simulink library "outp"  (R2021b)
(part 11 of 11)

  VTPM_WriteChkLFID_raw/1 -> VTPM_WriteChkLFID_raw_Inproc/1  "VTPM_WriteChkLFID_raw"
  VTPM_WriteChkLFID_raw_Inproc/1 -> UnitConverter899/1
  UnitConverter899/1 -> VOUTP_WriteChkLFID_raw/1  "VOUTP_WriteChkLFID_raw"
  VTPM_WriteChkRFID_raw/1 -> VTPM_WriteChkRFID_raw_Inproc/1  "VTPM_WriteChkRFID_raw"
  VTPM_WriteChkRFID_raw_Inproc/1 -> UnitConverter900/1
  UnitConverter900/1 -> VOUTP_WriteChkRFID_raw/1  "VOUTP_WriteChkRFID_raw"
  VTPM_WriteChkLRID_raw/1 -> VTPM_WriteChkLRID_raw_Inproc/1  "VTPM_WriteChkLRID_raw"
  VTPM_WriteChkLRID_raw_Inproc/1 -> UnitConverter901/1
  UnitConverter901/1 -> VOUTP_WriteChkLRID_raw/1  "VOUTP_WriteChkLRID_raw"
  VTPM_WriteChkRRID_raw/1 -> VTPM_WriteChkRRID_raw_Inproc/1  "VTPM_WriteChkRRID_raw"
  VTPM_WriteChkRRID_raw_Inproc/1 -> UnitConverter902/1
  UnitConverter902/1 -> VOUTP_WriteChkRRID_raw/1  "VOUTP_WriteChkRRID_raw"
  VTPM_WriteChkfinLFID_raw/1 -> VTPM_WriteChkfinLFID_raw_Inproc/1  "VTPM_WriteChkfinLFID_raw"
  VTPM_WriteChkfinLFID_raw_Inproc/1 -> UnitConverter903/1
  UnitConverter903/1 -> VOUTP_WriteChkfinLFID_raw/1  "VOUTP_WriteChkfinLFID_raw"
  VTPM_WriteChkfinRFID_raw/1 -> VTPM_WriteChkfinRFID_raw_Inproc/1  "VTPM_WriteChkfinRFID_raw"
  VTPM_WriteChkfinRFID_raw_Inproc/1 -> UnitConverter904/1
  UnitConverter904/1 -> VOUTP_WriteChkfinRFID_raw/1  "VOUTP_WriteChkfinRFID_raw"
  VTPM_WriteChkfinLRID_raw/1 -> VTPM_WriteChkfinLRID_raw_Inproc/1  "VTPM_WriteChkfinLRID_raw"
  VTPM_WriteChkfinLRID_raw_Inproc/1 -> UnitConverter905/1
  UnitConverter905/1 -> VOUTP_WriteChkfinLRID_raw/1  "VOUTP_WriteChkfinLRID_raw"
  VTPM_WriteChkfinRRID_raw/1 -> VTPM_WriteChkfinRRID_raw_Inproc/1  "VTPM_WriteChkfinRRID_raw"
  VTPM_WriteChkfinRRID_raw_Inproc/1 -> UnitConverter906/1
  UnitConverter906/1 -> VOUTP_WriteChkfinRRID_raw/1  "VOUTP_WriteChkfinRRID_raw"
  VTPM_Flashchkdatavalid_enum/1 -> VTPM_Flashchkdatavalid_enum_Inproc/1  "VTPM_Flashchkdatavalid_enum"
  VTPM_Flashchkdatavalid_enum_Inproc/1 -> UnitConverter907/1
  UnitConverter907/1 -> VOUTP_Flashchkdatavalid_enum/1  "VOUTP_Flashchkdatavalid_enum"
  VTPM_Flashdatavalid_enum/1 -> VTPM_Flashdatavalid_enum_Inproc/1  "VTPM_Flashdatavalid_enum"
  VTPM_Flashdatavalid_enum_Inproc/1 -> UnitConverter908/1
  UnitConverter908/1 -> VOUTP_Flashdatavalid_enum/1  "VOUTP_Flashdatavalid_enum"
  VTPM_unlearnSfali_flg/1 -> VTPM_unlearnSfali_flg_Inproc/1  "VTPM_unlearnSfali_flg"
  VTPM_unlearnSfali_flg_Inproc/1 -> UnitConverter909/1
  UnitConverter909/1 -> VOUTP_unlearnSfali_flg/1  "VOUTP_unlearnSfali_flg"
  VTPM_unlearnSfailvalid_enum/1 -> VTPM_unlearnSfailvalid_enum_Inproc/1  "VTPM_unlearnSfailvalid_enum"
  VTPM_unlearnSfailvalid_enum_Inproc/1 -> UnitConverter910/1
  UnitConverter910/1 -> VOUTP_unlearnSfailvalid_enum/1  "VOUTP_unlearnSfailvalid_enum"
  VTPM_Prepresstempvalid_enum/1 -> VTPM_Prepresstempvalid_enum_Inproc/1  "VTPM_Prepresstempvalid_enum"
  VTPM_Prepresstempvalid_enum_Inproc/1 -> UnitConverter911/1
  UnitConverter911/1 -> VOUTP_Prepresstempvalid_enum/1  "VOUTP_Prepresstempvalid_enum"
  VTPM_FlashS1ID_raw/1 -> VTPM_FlashS1ID_raw_Inproc/1  "VTPM_FlashS1ID_raw"
  VTPM_FlashS1ID_raw_Inproc/1 -> UnitConverter912/1
  UnitConverter912/1 -> VOUTP_FlashS1ID_raw/1  "VOUTP_FlashS1ID_raw"
  VTPM_FlashS2ID_raw/1 -> VTPM_FlashS2ID_raw_Inproc/1  "VTPM_FlashS2ID_raw"
  VTPM_FlashS2ID_raw_Inproc/1 -> UnitConverter913/1
  UnitConverter913/1 -> VOUTP_FlashS2ID_raw/1  "VOUTP_FlashS2ID_raw"
  VTPM_FlashS3ID_raw/1 -> VTPM_FlashS3ID_raw_Inproc/1  "VTPM_FlashS3ID_raw"
  VTPM_FlashS3ID_raw_Inproc/1 -> UnitConverter914/1
  UnitConverter914/1 -> VOUTP_FlashS3ID_raw/1  "VOUTP_FlashS3ID_raw"
  VTPM_FlashS4ID_raw/1 -> VTPM_FlashS4ID_raw_Inproc/1  "VTPM_FlashS4ID_raw"
  VTPM_FlashS4ID_raw_Inproc/1 -> UnitConverter915/1
  UnitConverter915/1 -> VOUTP_FlashS4ID_raw/1  "VOUTP_FlashS4ID_raw"
  VTPM_FlashIDvalid_enum/1 -> VTPM_FlashIDvalid_enum_Inproc/1  "VTPM_FlashIDvalid_enum"
  VTPM_FlashIDvalid_enum_Inproc/1 -> UnitConverter916/1
  UnitConverter916/1 -> VOUTP_FlashIDvalid_enum/1  "VOUTP_FlashIDvalid_enum"
  VTPM_WritingCnt_enum/1 -> VTPM_WritingCnt_enum_Inproc/1  "VTPM_WritingCnt_enum"
  VTPM_WritingCnt_enum_Inproc/1 -> UnitConverter917/1
  UnitConverter917/1 -> VOUTP_WritingCnt_enum/1  "VOUTP_WritingCnt_enum"
  VTPM_TPMSTLCmd_flg/1 -> VTPM_TPMSTLCmd_flg_Inproc/1  "VTPM_TPMSTLCmd_flg"
  VTPM_TPMSTLCmd_flg_Inproc/1 -> UnitConverter918/1
  UnitConverter918/1 -> VOUTP_TPMSTLCmd_flg/1  "VOUTP_TPMSTLCmd_flg"
  VTPM_LProgress_enum/1 -> VTPM_LProgress_enum_Inproc/1  "VTPM_LProgress_enum"
  VTPM_LProgress_enum_Inproc/1 -> UnitConverter919/1
  UnitConverter919/1 -> VOUTP_LProgress_enum/1  "VOUTP_LProgress_enum"
  VTPM_TPMSSensorIDRegStart_flg/1 -> VTPM_TPMSSensorIDRegStart_flg_Inproc/1  "VTPM_TPMSSensorIDRegStart_flg"
  VTPM_TPMSSensorIDRegStart_flg_Inproc/1 -> UnitConverter920/1
  UnitConverter920/1 -> VOUTP_TPMSSensorIDRegStart_flg/1  "VOUTP_TPMSSensorIDRegStart_flg"
  VTPM_ModelVersion_raw/1 -> VTPM_ModelVersion_raw_Inproc/1  "VTPM_ModelVersion_raw"
  VTPM_ModelVersion_raw_Inproc/1 -> UnitConverter921/1
  UnitConverter921/1 -> VOUTP_ModelVersion_raw/1  "VOUTP_ModelVersion_raw"
  VTPM_ModelVersionChksum_raw/1 -> VTPM_ModelVersionChksum_raw_Inproc/1  "VTPM_ModelVersionChksum_raw"
  VTPM_ModelVersionChksum_raw_Inproc/1 -> UnitConverter922/1
  UnitConverter922/1 -> VOUTP_ModelVersionChksum_raw/1  "VOUTP_ModelVersionChksum_raw"
  VTQD_ParkRequest_flg/1 -> VTQD_ParkRequest_flg_Inproc/1  "VTQD_ParkRequest_flg"
  VTQD_ParkRequest_flg_Inproc/1 -> UnitConverter923/1
  UnitConverter923/1 -> VOUTP_ParkRequest_flg/1  "VOUTP_ParkRequest_flg"
  VTQD_TqSourceFr_enum/1 -> VTQD_TqSourceFr_enum_Inproc/1  "VTQD_TqSourceFr_enum"
  VTQD_TqSourceFr_enum_Inproc/1 -> UnitConverter924/1
  UnitConverter924/1 -> VOUTP_TqSourceFr_enum/1  "VOUTP_TqSourceFr_enum"
  VTQD_TqSourceRr_enum/1 -> VTQD_TqSourceRr_enum_Inproc/1  "VTQD_TqSourceRr_enum"
  VTQD_TqSourceRr_enum_Inproc/1 -> UnitConverter925/1
  UnitConverter925/1 -> VOUTP_TqSourceRr_enum/1  "VOUTP_TqSourceRr_enum"
  VTQD_FrEDUAvailBrkRgnTq_Nm/1 -> VTQD_FrEDUAvailBrkRgnTq_Nm_Inproc/1  "VTQD_FrEDUAvailBrkRgnTq_Nm"
  VTQD_FrEDUAvailBrkRgnTq_Nm_Inproc/1 -> UnitConverter926/1
  UnitConverter926/1 -> VOUTP_FrEDUAvailBrkRgnTq_Nm/1  "VOUTP_FrEDUAvailBrkRgnTq_Nm"
  VTQD_RrEDUAvailBrkRgnTq_Nm/1 -> VTQD_RrEDUAvailBrkRgnTq_Nm_Inproc/1  "VTQD_RrEDUAvailBrkRgnTq_Nm"
  VTQD_RrEDUAvailBrkRgnTq_Nm_Inproc/1 -> UnitConverter927/1
  UnitConverter927/1 -> VOUTP_RrEDUAvailBrkRgnTq_Nm/1  "VOUTP_RrEDUAvailBrkRgnTq_Nm"
  VTQD_EVDriveMode_enum/1 -> VTQD_EVDriveMode_enum_Inproc/1  "VTQD_EVDriveMode_enum"
  VTQD_EVDriveMode_enum_Inproc/1 -> UnitConverter928/1
  UnitConverter928/1 -> VOUTP_EVDriveMode_enum/1  "VOUTP_EVDriveMode_enum"
  VTQD_ShiftGearPosn_enum/1 -> VTQD_ShiftGearPosn_enum_Inproc/1  "VTQD_ShiftGearPosn_enum"
  VTQD_ShiftGearPosn_enum_Inproc/1 -> UnitConverter929/1
  UnitConverter929/1 -> VOUTP_ShiftGearPosn_enum/1  "VOUTP_ShiftGearPosn_enum"
  VTQD_PButtonSta_enum/1 -> VTQD_PButtonSta_enum_Inproc/1  "VTQD_PButtonSta_enum"
  VTQD_PButtonSta_enum_Inproc/1 -> UnitConverter930/1
  UnitConverter930/1 -> VOUTP_PButtonSta_enum/1  "VOUTP_PButtonSta_enum"
  VTQD_FrActvDmpDisabReq_flg/1 -> VTQD_FrActvDmpDisabReq_flg_Inproc/1  "VTQD_FrActvDmpDisabReq_flg"
  VTQD_FrActvDmpDisabReq_flg_Inproc/1 -> UnitConverter931/1
  UnitConverter931/1 -> VOUTP_FrActvDmpDisabReq_flg/1  "VOUTP_FrActvDmpDisabReq_flg"
  VTQD_RrActvDmpDisabReq_flg/1 -> VTQD_RrActvDmpDisabReq_flg_Inproc/1  "VTQD_RrActvDmpDisabReq_flg"
  VTQD_RrActvDmpDisabReq_flg_Inproc/1 -> UnitConverter932/1
  UnitConverter932/1 -> VOUTP_RrActvDmpDisabReq_flg/1  "VOUTP_RrActvDmpDisabReq_flg"
  VTQD_FrRgnDecrSta_flg/1 -> VTQD_FrRgnDecrSta_flg_Inproc/1  "VTQD_FrRgnDecrSta_flg"
  VTQD_FrRgnDecrSta_flg_Inproc/1 -> UnitConverter933/1
  UnitConverter933/1 -> VOUTP_FrRgnDecrSta_flg/1  "VOUTP_FrRgnDecrSta_flg"
  VTQD_RrRgnDecrSta_flg/1 -> VTQD_RrRgnDecrSta_flg_Inproc/1  "VTQD_RrRgnDecrSta_flg"
  VTQD_RrRgnDecrSta_flg_Inproc/1 -> UnitConverter934/1
  UnitConverter934/1 -> VOUTP_RrRgnDecrSta_flg/1  "VOUTP_RrRgnDecrSta_flg"
  VTQD_DriverWhlTqDemFr_Nm/1 -> VTQD_DriverWhlTqDemFr_Nm_Inproc/1  "VTQD_DriverWhlTqDemFr_Nm"
  VTQD_DriverWhlTqDemFr_Nm_Inproc/1 -> UnitConverter935/1
  UnitConverter935/1 -> VOUTP_DriverWhlTqDemFr_Nm/1  "VOUTP_DriverWhlTqDemFr_Nm"
  VTQD_DriverWhlTqDemRr_Nm/1 -> VTQD_DriverWhlTqDemRr_Nm_Inproc/1  "VTQD_DriverWhlTqDemRr_Nm"
  VTQD_DriverWhlTqDemRr_Nm_Inproc/1 -> UnitConverter936/1
  UnitConverter936/1 -> VOUTP_DriverWhlTqDemRr_Nm/1  "VOUTP_DriverWhlTqDemRr_Nm"
  VTQD_FrEDUActTq_Nm/1 -> VTQD_FrEDUActTq_Nm_Inproc/1  "VTQD_FrEDUActTq_Nm"
  VTQD_FrEDUActTq_Nm_Inproc/1 -> UnitConverter937/1
  UnitConverter937/1 -> VOUTP_FrEDUActTq_Nm/1  "VOUTP_FrEDUActTq_Nm"
  VTQD_RrEDUActTq_Nm/1 -> VTQD_RrEDUActTq_Nm_Inproc/1  "VTQD_RrEDUActTq_Nm"
  VTQD_RrEDUActTq_Nm_Inproc/1 -> UnitConverter938/1
  UnitConverter938/1 -> VOUTP_RrEDUActTq_Nm/1  "VOUTP_RrEDUActTq_Nm"
  VTQD_FrEDURolRgnTq_Nm/1 -> VTQD_FrEDURolRgnTq_Nm_Inproc/1  "VTQD_FrEDURolRgnTq_Nm"
  VTQD_FrEDURolRgnTq_Nm_Inproc/1 -> UnitConverter939/1
  UnitConverter939/1 -> VOUTP_FrEDURolRgnTq_Nm/1  "VOUTP_FrEDURolRgnTq_Nm"
  VTQD_RrEDURolRgnTq_Nm/1 -> VTQD_RrEDURolRgnTq_Nm_Inproc/1  "VTQD_RrEDURolRgnTq_Nm"
  VTQD_RrEDURolRgnTq_Nm_Inproc/1 -> UnitConverter940/1
  UnitConverter940/1 -> VOUTP_RrEDURolRgnTq_Nm/1  "VOUTP_RrEDURolRgnTq_Nm"
  VTQD_FrEDUSpd_rpm/1 -> VTQD_FrEDUSpd_rpm_Inproc/1  "VTQD_FrEDUSpd_rpm"
  VTQD_FrEDUSpd_rpm_Inproc/1 -> UnitConverter941/1
  UnitConverter941/1 -> VOUTP_FrEDUSpd_rpm/1  "VOUTP_FrEDUSpd_rpm"
  VTQD_RrEDUSpd_rpm/1 -> VTQD_RrEDUSpd_rpm_Inproc/1  "VTQD_RrEDUSpd_rpm"
  VTQD_RrEDUSpd_rpm_Inproc/1 -> UnitConverter942/1
  UnitConverter942/1 -> VOUTP_RrEDUSpd_rpm/1  "VOUTP_RrEDUSpd_rpm"
  VTQD_FrEDUSpdValid_flg/1 -> VTQD_FrEDUSpdValid_flg_Inproc/1  "VTQD_FrEDUSpdValid_flg"
  VTQD_FrEDUSpdValid_flg_Inproc/1 -> UnitConverter943/1
  UnitConverter943/1 -> VOUTP_FrEDUSpdValid_flg/1  "VOUTP_FrEDUSpdValid_flg"
  VTQD_FrEDUAvailBrkRgnTqV_flg/1 -> VTQD_FrEDUAvailBrkRgnTqV_flg_Inproc/1  "VTQD_FrEDUAvailBrkRgnTqV_flg"
  VTQD_FrEDUAvailBrkRgnTqV_flg_Inproc/1 -> UnitConverter944/1
  UnitConverter944/1 -> VOUTP_FrEDUAvailBrkRgnTqV_flg/1  "VOUTP_FrEDUAvailBrkRgnTqV_flg"
  VTQD_RrEDUSpdValid_flg/1 -> VTQD_RrEDUSpdValid_flg_Inproc/1  "VTQD_RrEDUSpdValid_flg"
  VTQD_RrEDUSpdValid_flg_Inproc/1 -> UnitConverter945/1
  UnitConverter945/1 -> VOUTP_RrEDUSpdValid_flg/1  "VOUTP_RrEDUSpdValid_flg"
  VTQD_RrEDUAvailBrkRgnTqV_flg/1 -> VTQD_RrEDUAvailBrkRgnTqV_flg_Inproc/1  "VTQD_RrEDUAvailBrkRgnTqV_flg"
  VTQD_RrEDUAvailBrkRgnTqV_flg_Inproc/1 -> UnitConverter946/1
  UnitConverter946/1 -> VOUTP_RrEDUAvailBrkRgnTqV_flg/1  "VOUTP_RrEDUAvailBrkRgnTqV_flg"
  VTQD_RgnAbnorSta_flg/1 -> VTQD_RgnAbnorSta_flg_Inproc/1  "VTQD_RgnAbnorSta_flg"
  VTQD_RgnAbnorSta_flg_Inproc/1 -> UnitConverter947/1
  UnitConverter947/1 -> VOUTP_RgnAbnorSta_flg/1  "VOUTP_RgnAbnorSta_flg"
  VTQD_PTCSPermSta_flg/1 -> VTQD_PTCSPermSta_flg_Inproc/1  "VTQD_PTCSPermSta_flg"
  VTQD_PTCSPermSta_flg_Inproc/1 -> UnitConverter948/1
  UnitConverter948/1 -> VOUTP_PTCSPermSta_flg/1  "VOUTP_PTCSPermSta_flg"
  VTQD_FrRgnPermSta_flg/1 -> VTQD_FrRgnPermSta_flg_Inproc/1  "VTQD_FrRgnPermSta_flg"
  VTQD_FrRgnPermSta_flg_Inproc/1 -> UnitConverter949/1
  UnitConverter949/1 -> VOUTP_FrRgnPermSta_flg/1  "VOUTP_FrRgnPermSta_flg"
  VTQD_RrRgnPermSta_flg/1 -> VTQD_RrRgnPermSta_flg_Inproc/1  "VTQD_RrRgnPermSta_flg"
  VTQD_RrRgnPermSta_flg_Inproc/1 -> UnitConverter950/1
  UnitConverter950/1 -> VOUTP_RrRgnPermSta_flg/1  "VOUTP_RrRgnPermSta_flg"
  VTQD_FrIdcMin_A/1 -> VTQD_FrIdcMin_A_Inproc/1  "VTQD_FrIdcMin_A"
  VTQD_FrIdcMin_A_Inproc/1 -> UnitConverter951/1
  UnitConverter951/1 -> VOUTP_FrIdcMin_A/1  "VOUTP_FrIdcMin_A"
  VTQD_FrIdcMax_A/1 -> VTQD_FrIdcMax_A_Inproc/1  "VTQD_FrIdcMax_A"
  VTQD_FrIdcMax_A_Inproc/1 -> UnitConverter952/1
  UnitConverter952/1 -> VOUTP_FrIdcMax_A/1  "VOUTP_FrIdcMax_A"
  VTQD_FrUdcMin_V/1 -> VTQD_FrUdcMin_V_Inproc/1  "VTQD_FrUdcMin_V"
  VTQD_FrUdcMin_V_Inproc/1 -> UnitConverter953/1
  UnitConverter953/1 -> VOUTP_FrUdcMin_V/1  "VOUTP_FrUdcMin_V"
  VTQD_FrUdcMax_V/1 -> VTQD_FrUdcMax_V_Inproc/1  "VTQD_FrUdcMax_V"
  VTQD_FrUdcMax_V_Inproc/1 -> UnitConverter954/1
  UnitConverter954/1 -> VOUTP_FrUdcMax_V/1  "VOUTP_FrUdcMax_V"
  VTQD_RrIdcMin_A/1 -> VTQD_RrIdcMin_A_Inproc/1  "VTQD_RrIdcMin_A"
  VTQD_RrIdcMin_A_Inproc/1 -> UnitConverter955/1
  UnitConverter955/1 -> VOUTP_RrIdcMin_A/1  "VOUTP_RrIdcMin_A"
  VTQD_RrIdcMax_A/1 -> VTQD_RrIdcMax_A_Inproc/1  "VTQD_RrIdcMax_A"
  VTQD_RrIdcMax_A_Inproc/1 -> UnitConverter956/1
  UnitConverter956/1 -> VOUTP_RrIdcMax_A/1  "VOUTP_RrIdcMax_A"
  VTQD_RrUdcMin_V/1 -> VTQD_RrUdcMin_V_Inproc/1  "VTQD_RrUdcMin_V"
  VTQD_RrUdcMin_V_Inproc/1 -> UnitConverter957/1
  UnitConverter957/1 -> VOUTP_RrUdcMin_V/1  "VOUTP_RrUdcMin_V"
  VTQD_RrUdcMax_V/1 -> VTQD_RrUdcMax_V_Inproc/1  "VTQD_RrUdcMax_V"
  VTQD_RrUdcMax_V_Inproc/1 -> UnitConverter958/1
  UnitConverter958/1 -> VOUTP_RrUdcMax_V/1  "VOUTP_RrUdcMax_V"
  VTQD_ReBrakeLPReq_flg/1 -> VTQD_ReBrakeLPReq_flg_Inproc/1  "VTQD_ReBrakeLPReq_flg"
  VTQD_ReBrakeLPReq_flg_Inproc/1 -> UnitConverter959/1
  UnitConverter959/1 -> VOUTP_ReBrakeLPReq_flg/1  "VOUTP_ReBrakeLPReq_flg"
  VTQD_CreepON_flg/1 -> VTQD_CreepON_flg_Inproc/1  "VTQD_CreepON_flg"
  VTQD_CreepON_flg_Inproc/1 -> UnitConverter960/1
  UnitConverter960/1 -> VOUTP_CreepON_flg/1  "VOUTP_CreepON_flg"
  VTQD_EquivAccPedalSWSta_flg/1 -> VTQD_EquivAccPedalSWSta_flg_Inproc/1  "VTQD_EquivAccPedalSWSta_flg"
  VTQD_EquivAccPedalSWSta_flg_Inproc/1 -> UnitConverter961/1
  UnitConverter961/1 -> VOUTP_EquivAccPedalSWSta_flg/1  "VOUTP_EquivAccPedalSWSta_flg"
  VTQD_DriveProtEn_flg/1 -> VTQD_DriveProtEn_flg_Inproc/1  "VTQD_DriveProtEn_flg"
  VTQD_DriveProtEn_flg_Inproc/1 -> UnitConverter962/1
  UnitConverter962/1 -> VOUTP_DriveProtEn_flg/1  "VOUTP_DriveProtEn_flg"
  VTQD_ActParkRequest_flg/1 -> VTQD_ActParkRequest_flg_Inproc/1  "VTQD_ActParkRequest_flg"
  VTQD_ActParkRequest_flg_Inproc/1 -> UnitConverter963/1
  UnitConverter963/1 -> VOUTP_ActParkRequest_flg/1  "VOUTP_ActParkRequest_flg"
  VTQD_IVIPwrLockSta_enum/1 -> VTQD_IVIPwrLockSta_enum_Inproc/1  "VTQD_IVIPwrLockSta_enum"
  VTQD_IVIPwrLockSta_enum_Inproc/1 -> UnitConverter964/1
  UnitConverter964/1 -> VOUTP_IVIPwrLockSta_enum/1  "VOUTP_IVIPwrLockSta_enum"
  VTQD_OPDHoldLamp_flg/1 -> VTQD_OPDHoldLamp_flg_Inproc/1  "VTQD_OPDHoldLamp_flg"
  VTQD_OPDHoldLamp_flg_Inproc/1 -> UnitConverter965/1
  UnitConverter965/1 -> VOUTP_OPDHoldLamp_flg/1  "VOUTP_OPDHoldLamp_flg"
  VTQD_SaveRegenMode_enum/1 -> VTQD_SaveRegenMode_enum_Inproc/1  "VTQD_SaveRegenMode_enum"
  VTQD_SaveRegenMode_enum_Inproc/1 -> UnitConverter966/1
  UnitConverter966/1 -> VOUTP_SaveRegenMode_enum/1  "VOUTP_SaveRegenMode_enum"
  VTQD_FDCVCURegenMode_enum/1 -> VTQD_FDCVCURegenMode_enum_Inproc/1  "VTQD_FDCVCURegenMode_enum"
  VTQD_FDCVCURegenMode_enum_Inproc/1 -> UnitConverter967/1
  UnitConverter967/1 -> VOUTP_FDCVCURegenMode_enum/1  "VOUTP_FDCVCURegenMode_enum"
  VTQD_SpdCtrlMode_enum/1 -> VTQD_SpdCtrlMode_enum_Inproc/1  "VTQD_SpdCtrlMode_enum"
  VTQD_SpdCtrlMode_enum_Inproc/1 -> UnitConverter968/1
  UnitConverter968/1 -> VOUTP_SpdCtrlMode_enum/1  "VOUTP_SpdCtrlMode_enum"
  VTQD_SpdCtrlSta_flg/1 -> VTQD_SpdCtrlSta_flg_Inproc/1  "VTQD_SpdCtrlSta_flg"
  VTQD_SpdCtrlSta_flg_Inproc/1 -> UnitConverter969/1
  UnitConverter969/1 -> VOUTP_SpdCtrlSta_flg/1  "VOUTP_SpdCtrlSta_flg"
  VTQD_SetSpd_kph/1 -> VTQD_SetSpd_kph_Inproc/1  "VTQD_SetSpd_kph"
  VTQD_SetSpd_kph_Inproc/1 -> UnitConverter970/1
  UnitConverter970/1 -> VOUTP_SetSpd_kph/1  "VOUTP_SetSpd_kph"
  VTQD_VehActSpd_kph/1 -> VTQD_VehActSpd_kph_Inproc/1  "VTQD_VehActSpd_kph"
  VTQD_VehActSpd_kph_Inproc/1 -> UnitConverter971/1
  UnitConverter971/1 -> VOUTP_VehActSpd_kph/1  "VOUTP_VehActSpd_kph"
  VTQD_RegenLimIndSta_flg/1 -> VTQD_RegenLimIndSta_flg_Inproc/1  "VTQD_RegenLimIndSta_flg"
  VTQD_RegenLimIndSta_flg_Inproc/1 -> UnitConverter972/1
  UnitConverter972/1 -> VOUTP_RegenLimIndSta_flg/1  "VOUTP_RegenLimIndSta_flg"
  VTQD_SetSpdLimWarn_flg/1 -> VTQD_SetSpdLimWarn_flg_Inproc/1  "VTQD_SetSpdLimWarn_flg"
  VTQD_SetSpdLimWarn_flg_Inproc/1 -> UnitConverter973/1
  UnitConverter973/1 -> VOUTP_SetSpdLimWarn_flg/1  "VOUTP_SetSpdLimWarn_flg"
  VTQR_FrTMTqReq_Nm/1 -> VTQR_FrTMTqReq_Nm_Inproc/1  "VTQR_FrTMTqReq_Nm"
  VTQR_FrTMTqReq_Nm_Inproc/1 -> UnitConverter974/1
  UnitConverter974/1 -> VOUTP_FrTMTqReq_Nm/1  "VOUTP_FrTMTqReq_Nm"
  VTQR_RrTMTqReq_Nm/1 -> VTQR_RrTMTqReq_Nm_Inproc/1  "VTQR_RrTMTqReq_Nm"
  VTQR_RrTMTqReq_Nm_Inproc/1 -> UnitConverter975/1
  UnitConverter975/1 -> VOUTP_RrTMTqReq_Nm/1  "VOUTP_RrTMTqReq_Nm"
  VV2L_ReqOBCV2LEna_enum/1 -> VV2L_ReqOBCV2LEna_enum_Inproc/1  "VV2L_ReqOBCV2LEna_enum"
  VV2L_ReqOBCV2LEna_enum_Inproc/1 -> UnitConverter976/1
  UnitConverter976/1 -> VOUTP_ReqOBCV2LEna_enum/1  "VOUTP_ReqOBCV2LEna_enum"
  VV2L_ReqV2LIVIPopup_enum/1 -> VV2L_ReqV2LIVIPopup_enum_Inproc/1  "VV2L_ReqV2LIVIPopup_enum"
  VV2L_ReqV2LIVIPopup_enum_Inproc/1 -> UnitConverter977/1
  UnitConverter977/1 -> VOUTP_ReqV2LIVIPopup_enum/1  "VOUTP_ReqV2LIVIPopup_enum"
  VV2L_ReqV2LIVIDisChrg_enum/1 -> VV2L_ReqV2LIVIDisChrg_enum_Inproc/1  "VV2L_ReqV2LIVIDisChrg_enum"
  VV2L_ReqV2LIVIDisChrg_enum_Inproc/1 -> UnitConverter978/1
  UnitConverter978/1 -> VOUTP_ReqV2LIVIDisChrg_enum/1  "VOUTP_ReqV2LIVIDisChrg_enum"
  VV2L_ReqOBCExtrV2LEna_enum/1 -> VV2L_ReqOBCExtrV2LEna_enum_Inproc/1  "VV2L_ReqOBCExtrV2LEna_enum"
  VV2L_ReqOBCExtrV2LEna_enum_Inproc/1 -> UnitConverter979/1
  UnitConverter979/1 -> VOUTP_ReqOBCExtrV2LEna_enum/1  "VOUTP_ReqOBCExtrV2LEna_enum"
  VV2L_ReqOBCIntrV2LEna_enum/1 -> VV2L_ReqOBCIntrV2LEna_enum_Inproc/1  "VV2L_ReqOBCIntrV2LEna_enum"
  VV2L_ReqOBCIntrV2LEna_enum_Inproc/1 -> UnitConverter980/1
  UnitConverter980/1 -> VOUTP_ReqOBCIntrV2LEna_enum/1  "VOUTP_ReqOBCIntrV2LEna_enum"
  VV2L_HVPO120VGrpALDSt_enum/1 -> VV2L_HVPO120VGrpALDSt_enum_Inproc/1  "VV2L_HVPO120VGrpALDSt_enum"
  VV2L_HVPO120VGrpALDSt_enum_Inproc/1 -> UnitConverter981/1
  UnitConverter981/1 -> VOUTP_HVPO120VGrpALDSt_enum/1  "VOUTP_HVPO120VGrpALDSt_enum"
  VV2L_HVPO120VGrpBLDSt_enum/1 -> VV2L_HVPO120VGrpBLDSt_enum_Inproc/1  "VV2L_HVPO120VGrpBLDSt_enum"
  VV2L_HVPO120VGrpBLDSt_enum_Inproc/1 -> UnitConverter982/1
  UnitConverter982/1 -> VOUTP_HVPO120VGrpBLDSt_enum/1  "VOUTP_HVPO120VGrpBLDSt_enum"
  VVMC_FeatSetSpdFinal_raw32/1 -> VVMC_FeatSetSpdFinal_raw32_Inproc/1  "VVMC_FeatSetSpdFinal_raw32"
  VVMC_FeatSetSpdFinal_raw32_Inproc/1 -> UnitConverter983/1
  UnitConverter983/1 -> VOUTP_FeatSetSpdFinal_raw32/1  "VOUTP_FeatSetSpdFinal_raw32"
  VVMC_VehicleSpeed_mph/1 -> VVMC_VehicleSpeed_mph_Inproc/1  "VVMC_VehicleSpeed_mph"
  VVMC_VehicleSpeed_mph_Inproc/1 -> UnitConverter984/1
  UnitConverter984/1 -> VOUTP_VehicleSpeed_mph/1  "VOUTP_VehicleSpeed_mph"
  VVMC_VehicleSpeed_kph/1 -> VVMC_VehicleSpeed_kph_Inproc/1  "VVMC_VehicleSpeed_kph"
  VVMC_VehicleSpeed_kph_Inproc/1 -> UnitConverter985/1
  UnitConverter985/1 -> VOUTP_VehicleSpeed_kph/1  "VOUTP_VehicleSpeed_kph"
  VVMC_MeterIndSpeed_raw32/1 -> VVMC_MeterIndSpeed_raw32_Inproc/1  "VVMC_MeterIndSpeed_raw32"
  VVMC_MeterIndSpeed_raw32_Inproc/1 -> UnitConverter986/1
  UnitConverter986/1 -> VOUTP_MeterIndSpeed_raw32/1  "VOUTP_MeterIndSpeed_raw32"
  VVMC_VMCAEBCtrlAvail_flg/1 -> VVMC_VMCAEBCtrlAvail_flg_Inproc/1  "VVMC_VMCAEBCtrlAvail_flg"
  VVMC_VMCAEBCtrlAvail_flg_Inproc/1 -> UnitConverter987/1
  UnitConverter987/1 -> VOUTP_VMCAEBCtrlAvail_flg/1  "VOUTP_VMCAEBCtrlAvail_flg"
  VVMC_VMCACCCtrlAvail_flg/1 -> VVMC_VMCACCCtrlAvail_flg_Inproc/1  "VVMC_VMCACCCtrlAvail_flg"
  VVMC_VMCACCCtrlAvail_flg_Inproc/1 -> UnitConverter988/1
  UnitConverter988/1 -> VOUTP_VMCACCCtrlAvail_flg/1  "VOUTP_VMCACCCtrlAvail_flg"
  VVMC_VMCCCCtrlAvail_flg/1 -> VVMC_VMCCCCtrlAvail_flg_Inproc/1  "VVMC_VMCCCCtrlAvail_flg"
  VVMC_VMCCCCtrlAvail_flg_Inproc/1 -> UnitConverter989/1
  UnitConverter989/1 -> VOUTP_VMCCCCtrlAvail_flg/1  "VOUTP_VMCCCCtrlAvail_flg"
  VVMC_VMCMSACtrlAvail_flg/1 -> VVMC_VMCMSACtrlAvail_flg_Inproc/1  "VVMC_VMCMSACtrlAvail_flg"
  VVMC_VMCMSACtrlAvail_flg_Inproc/1 -> UnitConverter990/1
  UnitConverter990/1 -> VOUTP_VMCMSACtrlAvail_flg/1  "VOUTP_VMCMSACtrlAvail_flg"
  VVMC_FeatArbitrSta_enum/1 -> VVMC_FeatArbitrSta_enum_Inproc/1  "VVMC_FeatArbitrSta_enum"
  VVMC_FeatArbitrSta_enum_Inproc/1 -> UnitConverter991/1
  UnitConverter991/1 -> VOUTP_FeatArbitrSta_enum/1  "VOUTP_FeatArbitrSta_enum"
  VVMC_FeatReqSpd_kph/1 -> VVMC_FeatReqSpd_kph_Inproc/1  "VVMC_FeatReqSpd_kph"
  VVMC_FeatReqSpd_kph_Inproc/1 -> UnitConverter992/1
  UnitConverter992/1 -> VOUTP_FeatReqSpd_kph/1  "VOUTP_FeatReqSpd_kph"
  VVMC_JerkPCT_pct/1 -> VVMC_JerkPCT_pct_Inproc/1  "VVMC_JerkPCT_pct"
  VVMC_JerkPCT_pct_Inproc/1 -> UnitConverter993/1
  UnitConverter993/1 -> VOUTP_JerkPCT_pct/1  "VOUTP_JerkPCT_pct"
  VVMC_LimitPCT_pct/1 -> VVMC_LimitPCT_pct_Inproc/1  "VVMC_LimitPCT_pct"
  VVMC_LimitPCT_pct_Inproc/1 -> UnitConverter994/1
  UnitConverter994/1 -> VOUTP_LimitPCT_pct/1  "VOUTP_LimitPCT_pct"
  VVMC_FrontRearSlipRatioCtrl_flg/1 -> VVMC_FrontRearSlipRatioCtrl_flg_Inproc/1  "VVMC_FrontRearSlipRatioCtrl_flg"
  VVMC_FrontRearSlipRatioCtrl_flg_Inproc/1 -> UnitConverter995/1
  UnitConverter995/1 -> VOUTP_FrontRearSlipRatioCtrl_flg/1  "VOUTP_FrontRearSlipRatioCtrl_flg"
  VVMC_RearWhlSlipRatioCtrl_flg/1 -> VVMC_RearWhlSlipRatioCtrl_flg_Inproc/1  "VVMC_RearWhlSlipRatioCtrl_flg"
  VVMC_RearWhlSlipRatioCtrl_flg_Inproc/1 -> UnitConverter996/1
  UnitConverter996/1 -> VOUTP_RearWhlSlipRatioCtrl_flg/1  "VOUTP_RearWhlSlipRatioCtrl_flg"
  VVMC_SingleWhlSlipRatioCtrl_flg/1 -> VVMC_SingleWhlSlipRatioCtrl_flg_Inproc/1  "VVMC_SingleWhlSlipRatioCtrl_flg"
  VVMC_SingleWhlSlipRatioCtrl_flg_Inproc/1 -> UnitConverter997/1
  UnitConverter997/1 -> VOUTP_SingleWhlSlipRatioCtrl_flg/1  "VOUTP_SingleWhlSlipRatioCtrl_flg"
  VVMC_LatAccCtrl_flg/1 -> VVMC_LatAccCtrl_flg_Inproc/1  "VVMC_LatAccCtrl_flg"
  VVMC_LatAccCtrl_flg_Inproc/1 -> UnitConverter998/1
  UnitConverter998/1 -> VOUTP_LatAccCtrl_flg/1  "VOUTP_LatAccCtrl_flg"
  VVMC_SafetyCtrl_flg/1 -> VVMC_SafetyCtrl_flg_Inproc/1  "VVMC_SafetyCtrl_flg"
  VVMC_SafetyCtrl_flg_Inproc/1 -> UnitConverter999/1
  UnitConverter999/1 -> VOUTP_SafetyCtrl_flg/1  "VOUTP_SafetyCtrl_flg"
  VVMC_SPD2ACCAct_flg/1 -> VVMC_SPD2ACCAct_flg_Inproc/1  "VVMC_SPD2ACCAct_flg"
  VVMC_SPD2ACCAct_flg_Inproc/1 -> UnitConverter1000/1
  UnitConverter1000/1 -> VOUTP_SPD2ACCAct_flg/1  "VOUTP_SPD2ACCAct_flg"
  VVMC_AccCalcuPID_mps2/1 -> VVMC_AccCalcuPID_mps2_Inproc/1  "VVMC_AccCalcuPID_mps2"
  VVMC_AccCalcuPID_mps2_Inproc/1 -> UnitConverter1001/1
  UnitConverter1001/1 -> VOUTP_AccCalcuPID_mps2/1  "VOUTP_AccCalcuPID_mps2"
  VVMC_ISOAccLimit_mps2/1 -> VVMC_ISOAccLimit_mps2_Inproc/1  "VVMC_ISOAccLimit_mps2"
  VVMC_ISOAccLimit_mps2_Inproc/1 -> UnitConverter1002/1
  UnitConverter1002/1 -> VOUTP_ISOAccLimit_mps2/1  "VOUTP_ISOAccLimit_mps2"
  VVMC_ISODecLimit_mps2/1 -> VVMC_ISODecLimit_mps2_Inproc/1  "VVMC_ISODecLimit_mps2"
  VVMC_ISODecLimit_mps2_Inproc/1 -> UnitConverter1003/1
  UnitConverter1003/1 -> VOUTP_ISODecLimit_mps2/1  "VOUTP_ISODecLimit_mps2"
  VVMC_ISOJerkLimit_mps3/1 -> VVMC_ISOJerkLimit_mps3_Inproc/1  "VVMC_ISOJerkLimit_mps3"
  VVMC_ISOJerkLimit_mps3_Inproc/1 -> UnitConverter1004/1
  UnitConverter1004/1 -> VOUTP_ISOJerkLimit_mps3/1  "VOUTP_ISOJerkLimit_mps3"
  VVMC_ACCRequiredAccel_mps2/1 -> VVMC_ACCRequiredAccel_mps2_Inproc/1  "VVMC_ACCRequiredAccel_mps2"
  VVMC_ACCRequiredAccel_mps2_Inproc/1 -> UnitConverter1005/1
  UnitConverter1005/1 -> VOUTP_ACCRequiredAccel_mps2/1  "VOUTP_ACCRequiredAccel_mps2"
  VVMC_DISCReqAcc_mps2/1 -> VVMC_DISCReqAcc_mps2_Inproc/1  "VVMC_DISCReqAcc_mps2"
  VVMC_DISCReqAcc_mps2_Inproc/1 -> UnitConverter1006/1
  UnitConverter1006/1 -> VOUTP_DISCReqAcc_mps2/1  "VOUTP_DISCReqAcc_mps2"
  VVMC_FeatArbitrFinal_enum/1 -> VVMC_FeatArbitrFinal_enum_Inproc/1  "VVMC_FeatArbitrFinal_enum"
  VVMC_FeatArbitrFinal_enum_Inproc/1 -> UnitConverter1007/1
  UnitConverter1007/1 -> VOUTP_FeatArbitrFinal_enum/1  "VOUTP_FeatArbitrFinal_enum"
  VVMC_ActACCRequiredAccel_mps2/1 -> VVMC_ActACCRequiredAccel_mps2_Inproc/1  "VVMC_ActACCRequiredAccel_mps2"
  VVMC_ActACCRequiredAccel_mps2_Inproc/1 -> UnitConverter1008/1
  UnitConverter1008/1 -> VOUTP_ActACCRequiredAccel_mps2/1  "VOUTP_ActACCRequiredAccel_mps2"
  VVMC_LateralCtrl_flg/1 -> VVMC_LateralCtrl_flg_Inproc/1  "VVMC_LateralCtrl_flg"
  VVMC_LateralCtrl_flg_Inproc/1 -> UnitConverter1009/1
  UnitConverter1009/1 -> VOUTP_LateralCtrl_flg/1  "VOUTP_LateralCtrl_flg"
  VVMC_ADASLKASta_enum/1 -> VVMC_ADASLKASta_enum_Inproc/1  "VVMC_ADASLKASta_enum"
  VVMC_ADASLKASta_enum_Inproc/1 -> UnitConverter1010/1
  UnitConverter1010/1 -> VOUTP_ADASLKASta_enum/1  "VOUTP_ADASLKASta_enum"
  VVMC_LKAStrToqReq_Nm/1 -> VVMC_LKAStrToqReq_Nm_Inproc/1  "VVMC_LKAStrToqReq_Nm"
  VVMC_LKAStrToqReq_Nm_Inproc/1 -> UnitConverter1011/1
  UnitConverter1011/1 -> VOUTP_LKAStrToqReq_Nm/1  "VOUTP_LKAStrToqReq_Nm"
  VVMC_LKATOIFault_flg/1 -> VVMC_LKATOIFault_flg_Inproc/1  "VVMC_LKATOIFault_flg"
  VVMC_LKATOIFault_flg_Inproc/1 -> UnitConverter1012/1
  UnitConverter1012/1 -> VOUTP_LKATOIFault_flg/1  "VOUTP_LKATOIFault_flg"
  VVMC_LKATOIAct_enum/1 -> VVMC_LKATOIAct_enum_Inproc/1  "VVMC_LKATOIAct_enum"
  VVMC_LKATOIAct_enum_Inproc/1 -> UnitConverter1013/1
  UnitConverter1013/1 -> VOUTP_LKATOIAct_enum/1  "VOUTP_LKATOIAct_enum"
  VVMC_ADASAEBReq_enum/1 -> VVMC_ADASAEBReq_enum_Inproc/1  "VVMC_ADASAEBReq_enum"
  VVMC_ADASAEBReq_enum_Inproc/1 -> UnitConverter1014/1
  UnitConverter1014/1 -> VOUTP_ADASAEBReq_enum/1  "VOUTP_ADASAEBReq_enum"
  VVMC_ADASFaultSta_flg/1 -> VVMC_ADASFaultSta_flg_Inproc/1  "VVMC_ADASFaultSta_flg"
  VVMC_ADASFaultSta_flg_Inproc/1 -> UnitConverter1015/1
  UnitConverter1015/1 -> VOUTP_ADASFaultSta_flg/1  "VOUTP_ADASFaultSta_flg"
  VVMC_AEBVehHoldReq_flg/1 -> VVMC_AEBVehHoldReq_flg_Inproc/1  "VVMC_AEBVehHoldReq_flg"
  VVMC_AEBVehHoldReq_flg_Inproc/1 -> UnitConverter1016/1
  UnitConverter1016/1 -> VOUTP_AEBVehHoldReq_flg/1  "VOUTP_AEBVehHoldReq_flg"
  VVMC_ACCVehHoldReq_flg/1 -> VVMC_ACCVehHoldReq_flg_Inproc/1  "VVMC_ACCVehHoldReq_flg"
  VVMC_ACCVehHoldReq_flg_Inproc/1 -> UnitConverter1017/1
  UnitConverter1017/1 -> VOUTP_ACCVehHoldReq_flg/1  "VOUTP_ACCVehHoldReq_flg"
  VVMC_ADASDBSReq_enum/1 -> VVMC_ADASDBSReq_enum_Inproc/1  "VVMC_ADASDBSReq_enum"
  VVMC_ADASDBSReq_enum_Inproc/1 -> UnitConverter1018/1
  UnitConverter1018/1 -> VOUTP_ADASDBSReq_enum/1  "VOUTP_ADASDBSReq_enum"
  VVMC_ADASACCSta_enum/1 -> VVMC_ADASACCSta_enum_Inproc/1  "VVMC_ADASACCSta_enum"
  VVMC_ADASACCSta_enum_Inproc/1 -> UnitConverter1019/1
  UnitConverter1019/1 -> VOUTP_ADASACCSta_enum/1  "VOUTP_ADASACCSta_enum"
  VVMC_ACCObjDist_m/1 -> VVMC_ACCObjDist_m_Inproc/1  "VVMC_ACCObjDist_m"
  VVMC_ACCObjDist_m_Inproc/1 -> UnitConverter1020/1
  UnitConverter1020/1 -> VOUTP_ACCObjDist_m/1  "VOUTP_ACCObjDist_m"
  VVMC_ACCObjRelSpd_mps/1 -> VVMC_ACCObjRelSpd_mps_Inproc/1  "VVMC_ACCObjRelSpd_mps"
  VVMC_ACCObjRelSpd_mps_Inproc/1 -> UnitConverter1021/1
  UnitConverter1021/1 -> VOUTP_ACCObjRelSpd_mps/1  "VOUTP_ACCObjRelSpd_mps"
  VVMC_TimeGapLevel_enum/1 -> VVMC_TimeGapLevel_enum_Inproc/1  "VVMC_TimeGapLevel_enum"
  VVMC_TimeGapLevel_enum_Inproc/1 -> UnitConverter1022/1
  UnitConverter1022/1 -> VOUTP_TimeGapLevel_enum/1  "VOUTP_TimeGapLevel_enum"
  VVMC_ACCJerkUpperLimit_mps3/1 -> VVMC_ACCJerkUpperLimit_mps3_Inproc/1  "VVMC_ACCJerkUpperLimit_mps3"
  VVMC_ACCJerkUpperLimit_mps3_Inproc/1 -> UnitConverter1023/1
  UnitConverter1023/1 -> VOUTP_ACCJerkUpperLimit_mps3/1  "VOUTP_ACCJerkUpperLimit_mps3"
  VVMC_ACCComfortBandUpper_mps2/1 -> VVMC_ACCComfortBandUpper_mps2_Inproc/1  "VVMC_ACCComfortBandUpper_mps2"
  VVMC_ACCComfortBandUpper_mps2_Inproc/1 -> UnitConverter1024/1
  UnitConverter1024/1 -> VOUTP_ACCComfortBandUpper_mps2/1  "VOUTP_ACCComfortBandUpper_mps2"
  VVMC_ACCJerkLowerLimit_mps3/1 -> VVMC_ACCJerkLowerLimit_mps3_Inproc/1  "VVMC_ACCJerkLowerLimit_mps3"
  VVMC_ACCJerkLowerLimit_mps3_Inproc/1 -> UnitConverter1025/1
  UnitConverter1025/1 -> VOUTP_ACCJerkLowerLimit_mps3/1  "VOUTP_ACCJerkLowerLimit_mps3"
  VVMC_ACCComfortBandLower_mps2/1 -> VVMC_ACCComfortBandLower_mps2_Inproc/1  "VVMC_ACCComfortBandLower_mps2"
  VVMC_ACCComfortBandLower_mps2_Inproc/1 -> UnitConverter1026/1
  UnitConverter1026/1 -> VOUTP_ACCComfortBandLower_mps2/1  "VOUTP_ACCComfortBandLower_mps2"
  VVMC_ADASVehSpdLim_raw32/1 -> VVMC_ADASVehSpdLim_raw32_Inproc/1  "VVMC_ADASVehSpdLim_raw32"
  VVMC_ADASVehSpdLim_raw32_Inproc/1 -> UnitConverter1027/1
  UnitConverter1027/1 -> VOUTP_ADASVehSpdLim_raw32/1  "VOUTP_ADASVehSpdLim_raw32"
  VVMC_ADASShftPosnReqA_flg/1 -> VVMC_ADASShftPosnReqA_flg_Inproc/1  "VVMC_ADASShftPosnReqA_flg"
  VVMC_ADASShftPosnReqA_flg_Inproc/1 -> UnitConverter1028/1
  UnitConverter1028/1 -> VOUTP_ADASShftPosnReqA_flg/1  "VOUTP_ADASShftPosnReqA_flg"
  VVMC_ADASShftPosnReq_enum/1 -> VVMC_ADASShftPosnReq_enum_Inproc/1  "VVMC_ADASShftPosnReq_enum"
  VVMC_ADASShftPosnReq_enum_Inproc/1 -> UnitConverter1029/1
  UnitConverter1029/1 -> VOUTP_ADASShftPosnReq_enum/1  "VOUTP_ADASShftPosnReq_enum"
  VVMC_ADASForceIdle_flg/1 -> VVMC_ADASForceIdle_flg_Inproc/1  "VVMC_ADASForceIdle_flg"
  VVMC_ADASForceIdle_flg_Inproc/1 -> UnitConverter1030/1
  UnitConverter1030/1 -> VOUTP_ADASForceIdle_flg/1  "VOUTP_ADASForceIdle_flg"
  VVMC_HazardWarningReq_flg/1 -> VVMC_HazardWarningReq_flg_Inproc/1  "VVMC_HazardWarningReq_flg"
  VVMC_HazardWarningReq_flg_Inproc/1 -> UnitConverter1031/1
  UnitConverter1031/1 -> VOUTP_HazardWarningReq_flg/1  "VOUTP_HazardWarningReq_flg"
  VVMC_RightTurnLightReq_flg/1 -> VVMC_RightTurnLightReq_flg_Inproc/1  "VVMC_RightTurnLightReq_flg"
  VVMC_RightTurnLightReq_flg_Inproc/1 -> UnitConverter1032/1
  UnitConverter1032/1 -> VOUTP_RightTurnLightReq_flg/1  "VOUTP_RightTurnLightReq_flg"
  VVMC_LeftTurnLightReq_flg/1 -> VVMC_LeftTurnLightReq_flg_Inproc/1  "VVMC_LeftTurnLightReq_flg"
  VVMC_LeftTurnLightReq_flg_Inproc/1 -> UnitConverter1033/1
  UnitConverter1033/1 -> VOUTP_LeftTurnLightReq_flg/1  "VOUTP_LeftTurnLightReq_flg"
  VVMC_ADASFCWSta_enum/1 -> VVMC_ADASFCWSta_enum_Inproc/1  "VVMC_ADASFCWSta_enum"
  VVMC_ADASFCWSta_enum_Inproc/1 -> UnitConverter1034/1
  UnitConverter1034/1 -> VOUTP_ADASFCWSta_enum/1  "VOUTP_ADASFCWSta_enum"
  VVMC_ADASLDWSta_enum/1 -> VVMC_ADASLDWSta_enum_Inproc/1  "VVMC_ADASLDWSta_enum"
  VVMC_ADASLDWSta_enum_Inproc/1 -> UnitConverter1035/1
  UnitConverter1035/1 -> VOUTP_ADASLDWSta_enum/1  "VOUTP_ADASLDWSta_enum"
  VVMC_ADASFltWrnReq_flg/1 -> VVMC_ADASFltWrnReq_flg_Inproc/1  "VVMC_ADASFltWrnReq_flg"
  VVMC_ADASFltWrnReq_flg_Inproc/1 -> UnitConverter1036/1
  UnitConverter1036/1 -> VOUTP_ADASFltWrnReq_flg/1  "VOUTP_ADASFltWrnReq_flg"
  VVMC_ACCObjDstLvl_enum/1 -> VVMC_ACCObjDstLvl_enum_Inproc/1  "VVMC_ACCObjDstLvl_enum"
  VVMC_ACCObjDstLvl_enum_Inproc/1 -> UnitConverter1037/1
  UnitConverter1037/1 -> VOUTP_ACCObjDstLvl_enum/1  "VOUTP_ACCObjDstLvl_enum"
  VVMC_ForceLowBeam_enum/1 -> VVMC_ForceLowBeam_enum_Inproc/1  "VVMC_ForceLowBeam_enum"
  VVMC_ForceLowBeam_enum_Inproc/1 -> UnitConverter1038/1
  UnitConverter1038/1 -> VOUTP_ForceLowBeam_enum/1  "VOUTP_ForceLowBeam_enum"
  VVMC_ACCTakeoverReq_flg/1 -> VVMC_ACCTakeoverReq_flg_Inproc/1  "VVMC_ACCTakeoverReq_flg"
  VVMC_ACCTakeoverReq_flg_Inproc/1 -> UnitConverter1039/1
  UnitConverter1039/1 -> VOUTP_ACCTakeoverReq_flg/1  "VOUTP_ACCTakeoverReq_flg"
  VVMC_ADASWarningMsg_enum/1 -> VVMC_ADASWarningMsg_enum_Inproc/1  "VVMC_ADASWarningMsg_enum"
  VVMC_ADASWarningMsg_enum_Inproc/1 -> UnitConverter1040/1
  UnitConverter1040/1 -> VOUTP_ADASWarningMsg_enum/1  "VOUTP_ADASWarningMsg_enum"
  VVMC_ADASCAMSpdLim_enum/1 -> VVMC_ADASCAMSpdLim_enum_Inproc/1  "VVMC_ADASCAMSpdLim_enum"
  VVMC_ADASCAMSpdLim_enum_Inproc/1 -> UnitConverter1041/1
  UnitConverter1041/1 -> VOUTP_ADASCAMSpdLim_enum/1  "VOUTP_ADASCAMSpdLim_enum"
  VVMC_TargetType_enum/1 -> VVMC_TargetType_enum_Inproc/1  "VVMC_TargetType_enum"
  VVMC_TargetType_enum_Inproc/1 -> UnitConverter1042/1
  UnitConverter1042/1 -> VOUTP_TargetType_enum/1  "VOUTP_TargetType_enum"
  VVMC_ADASSLIFSpdLim_enum/1 -> VVMC_ADASSLIFSpdLim_enum_Inproc/1  "VVMC_ADASSLIFSpdLim_enum"
  VVMC_ADASSLIFSpdLim_enum_Inproc/1 -> UnitConverter1043/1
  UnitConverter1043/1 -> VOUTP_ADASSLIFSpdLim_enum/1  "VOUTP_ADASSLIFSpdLim_enum"
  VVMC_LKAHODDisplayWarning_flg/1 -> VVMC_LKAHODDisplayWarning_flg_Inproc/1  "VVMC_LKAHODDisplayWarning_flg"
  VVMC_LKAHODDisplayWarning_flg_Inproc/1 -> UnitConverter1044/1
  UnitConverter1044/1 -> VOUTP_LKAHODDisplayWarning_flg/1  "VOUTP_LKAHODDisplayWarning_flg"
  VVMC_LKAHODSoundWarning_flg/1 -> VVMC_LKAHODSoundWarning_flg_Inproc/1  "VVMC_LKAHODSoundWarning_flg"
  VVMC_LKAHODSoundWarning_flg_Inproc/1 -> UnitConverter1045/1
  UnitConverter1045/1 -> VOUTP_LKAHODSoundWarning_flg/1  "VOUTP_LKAHODSoundWarning_flg"
  VVMC_ADASLFCSta_enum/1 -> VVMC_ADASLFCSta_enum_Inproc/1  "VVMC_ADASLFCSta_enum"
  VVMC_ADASLFCSta_enum_Inproc/1 -> UnitConverter1046/1
  UnitConverter1046/1 -> VOUTP_ADASLFCSta_enum/1  "VOUTP_ADASLFCSta_enum"
  VVMC_ADASLaneModeL_enum/1 -> VVMC_ADASLaneModeL_enum_Inproc/1  "VVMC_ADASLaneModeL_enum"
  VVMC_ADASLaneModeL_enum_Inproc/1 -> UnitConverter1047/1
  UnitConverter1047/1 -> VOUTP_ADASLaneModeL_enum/1  "VOUTP_ADASLaneModeL_enum"
  VVMC_ADASLaneModeR_enum/1 -> VVMC_ADASLaneModeR_enum_Inproc/1  "VVMC_ADASLaneModeR_enum"
  VVMC_ADASLaneModeR_enum_Inproc/1 -> UnitConverter1048/1
  UnitConverter1048/1 -> VOUTP_ADASLaneModeR_enum/1  "VOUTP_ADASLaneModeR_enum"
  VVMC_ADASSLIFSta_enum/1 -> VVMC_ADASSLIFSta_enum_Inproc/1  "VVMC_ADASSLIFSta_enum"
  VVMC_ADASSLIFSta_enum_Inproc/1 -> UnitConverter1049/1
  UnitConverter1049/1 -> VOUTP_ADASSLIFSta_enum/1  "VOUTP_ADASSLIFSta_enum"
  VVMC_ADASISASta_enum/1 -> VVMC_ADASISASta_enum_Inproc/1  "VVMC_ADASISASta_enum"
  VVMC_ADASISASta_enum_Inproc/1 -> UnitConverter1050/1
  UnitConverter1050/1 -> VOUTP_ADASISASta_enum/1  "VOUTP_ADASISASta_enum"
  VVMC_ADASLDWMute_flg/1 -> VVMC_ADASLDWMute_flg_Inproc/1  "VVMC_ADASLDWMute_flg"
  VVMC_ADASLDWMute_flg_Inproc/1 -> UnitConverter1051/1
  UnitConverter1051/1 -> VOUTP_ADASLDWMute_flg/1  "VOUTP_ADASLDWMute_flg"
  VVMC_ADASFCWMute_flg/1 -> VVMC_ADASFCWMute_flg_Inproc/1  "VVMC_ADASFCWMute_flg"
  VVMC_ADASFCWMute_flg_Inproc/1 -> UnitConverter1052/1
  UnitConverter1052/1 -> VOUTP_ADASFCWMute_flg/1  "VOUTP_ADASFCWMute_flg"
  VVMC_ADASLFCHandsOffWarning_enum/1 -> VVMC_ADASLFCHandsOffWarning_enum_Inproc/1  "VVMC_ADASLFCHandsOffWarning_enum"
  VVMC_ADASLFCHandsOffWarning_enum_Inproc/1 -> UnitConverter1053/1
  UnitConverter1053/1 -> VOUTP_ADASLFCHandsOffWarning_enum/1  "VOUTP_ADASLFCHandsOffWarning_enum"
  VVMC_LVDADisabled_flg/1 -> VVMC_LVDADisabled_flg_Inproc/1  "VVMC_LVDADisabled_flg"
  VVMC_LVDADisabled_flg_Inproc/1 -> UnitConverter1054/1
  UnitConverter1054/1 -> VOUTP_LVDADisabled_flg/1  "VOUTP_LVDADisabled_flg"
  VVMC_LVDAMuteSta_enum/1 -> VVMC_LVDAMuteSta_enum_Inproc/1  "VVMC_LVDAMuteSta_enum"
  VVMC_LVDAMuteSta_enum_Inproc/1 -> UnitConverter1055/1
  UnitConverter1055/1 -> VOUTP_LVDAMuteSta_enum/1  "VOUTP_LVDAMuteSta_enum"
  VVMC_LVDAFailinfo_flg/1 -> VVMC_LVDAFailinfo_flg_Inproc/1  "VVMC_LVDAFailinfo_flg"
  VVMC_LVDAFailinfo_flg_Inproc/1 -> UnitConverter1056/1
  UnitConverter1056/1 -> VOUTP_LVDAFailinfo_flg/1  "VOUTP_LVDAFailinfo_flg"
  VVMC_LVDAWarning_flg/1 -> VVMC_LVDAWarning_flg_Inproc/1  "VVMC_LVDAWarning_flg"
  VVMC_LVDAWarning_flg_Inproc/1 -> UnitConverter1057/1
  UnitConverter1057/1 -> VOUTP_LVDAWarning_flg/1  "VOUTP_LVDAWarning_flg"
  VVMC_LVDAACCStatusInformation_flg/1 -> VVMC_LVDAACCStatusInformation_flg_Inproc/1  "VVMC_LVDAACCStatusInformation_flg"
  VVMC_LVDAACCStatusInformation_flg_Inproc/1 -> UnitConverter1058/1
  UnitConverter1058/1 -> VOUTP_LVDAACCStatusInformation_flg/1  "VOUTP_LVDAACCStatusInformation_flg"
  VVMC_ADASLFCWarnSound_enum/1 -> VVMC_ADASLFCWarnSound_enum_Inproc/1  "VVMC_ADASLFCWarnSound_enum"
  VVMC_ADASLFCWarnSound_enum_Inproc/1 -> UnitConverter1059/1
  UnitConverter1059/1 -> VOUTP_ADASLFCWarnSound_enum/1  "VOUTP_ADASLFCWarnSound_enum"
  VVMC_FCMACCmode_enum/1 -> VVMC_FCMACCmode_enum_Inproc/1  "VVMC_FCMACCmode_enum"
  VVMC_FCMACCmode_enum_Inproc/1 -> UnitConverter1060/1
  UnitConverter1060/1 -> VOUTP_FCMACCmode_enum/1  "VOUTP_FCMACCmode_enum"
  VVMC_ADASLanetypeR_enum/1 -> VVMC_ADASLanetypeR_enum_Inproc/1  "VVMC_ADASLanetypeR_enum"
  VVMC_ADASLanetypeR_enum_Inproc/1 -> UnitConverter1061/1
  UnitConverter1061/1 -> VOUTP_ADASLanetypeR_enum/1  "VOUTP_ADASLanetypeR_enum"
  VVMC_ADASLanetypeL_enum/1 -> VVMC_ADASLanetypeL_enum_Inproc/1  "VVMC_ADASLanetypeL_enum"
  VVMC_ADASLanetypeL_enum_Inproc/1 -> UnitConverter1062/1
  UnitConverter1062/1 -> VOUTP_ADASLanetypeL_enum/1  "VOUTP_ADASLanetypeL_enum"
  VVMC_ADASLanecurveL_raw32/1 -> VVMC_ADASLanecurveL_raw32_Inproc/1  "VVMC_ADASLanecurveL_raw32"
  VVMC_ADASLanecurveL_raw32_Inproc/1 -> UnitConverter1063/1
  UnitConverter1063/1 -> VOUTP_ADASLanecurveL_raw32/1  "VOUTP_ADASLanecurveL_raw32"
  VVMC_ADASLanecurveR_raw32/1 -> VVMC_ADASLanecurveR_raw32_Inproc/1  "VVMC_ADASLanecurveR_raw32"
  VVMC_ADASLanecurveR_raw32_Inproc/1 -> UnitConverter1064/1
  UnitConverter1064/1 -> VOUTP_ADASLanecurveR_raw32/1  "VOUTP_ADASLanecurveR_raw32"
  VVMC_ADASAEBSta_enum/1 -> VVMC_ADASAEBSta_enum_Inproc/1  "VVMC_ADASAEBSta_enum"
  VVMC_ADASAEBSta_enum_Inproc/1 -> UnitConverter1065/1
  UnitConverter1065/1 -> VOUTP_ADASAEBSta_enum/1  "VOUTP_ADASAEBSta_enum"
  VVMC_FCMLDWRequest_enum/1 -> VVMC_FCMLDWRequest_enum_Inproc/1  "VVMC_FCMLDWRequest_enum"
  VVMC_FCMLDWRequest_enum_Inproc/1 -> UnitConverter1066/1
  UnitConverter1066/1 -> VOUTP_FCMLDWRequest_enum/1  "VOUTP_FCMLDWRequest_enum"
  VVMC_FCMLDWFault_flg/1 -> VVMC_FCMLDWFault_flg_Inproc/1  "VVMC_FCMLDWFault_flg"
  VVMC_FCMLDWFault_flg_Inproc/1 -> UnitConverter1067/1
  UnitConverter1067/1 -> VOUTP_FCMLDWFault_flg/1  "VOUTP_FCMLDWFault_flg"
  VVMC_ACCCtrlAvail_flg/1 -> VVMC_ACCCtrlAvail_flg_Inproc/1  "VVMC_ACCCtrlAvail_flg"
  VVMC_ACCCtrlAvail_flg_Inproc/1 -> UnitConverter1068/1
  UnitConverter1068/1 -> VOUTP_ACCCtrlAvail_flg/1  "VOUTP_ACCCtrlAvail_flg"
  VVMC_ACCPedalOvrd_flg/1 -> VVMC_ACCPedalOvrd_flg_Inproc/1  "VVMC_ACCPedalOvrd_flg"
  VVMC_ACCPedalOvrd_flg_Inproc/1 -> UnitConverter1069/1
  UnitConverter1069/1 -> VOUTP_ACCPedalOvrd_flg/1  "VOUTP_ACCPedalOvrd_flg"
  VVMC_TimeGapCalcu_s/1 -> VVMC_TimeGapCalcu_s_Inproc/1  "VVMC_TimeGapCalcu_s"
  VVMC_TimeGapCalcu_s_Inproc/1 -> UnitConverter1070/1
  UnitConverter1070/1 -> VOUTP_TimeGapCalcu_s/1  "VOUTP_TimeGapCalcu_s"
  VVMC_CCCtrlSta_enum/1 -> VVMC_CCCtrlSta_enum_Inproc/1  "VVMC_CCCtrlSta_enum"
  VVMC_CCCtrlSta_enum_Inproc/1 -> UnitConverter1071/1
  UnitConverter1071/1 -> VOUTP_CCCtrlSta_enum/1  "VOUTP_CCCtrlSta_enum"
  VVMC_MSACtrlSta_enum/1 -> VVMC_MSACtrlSta_enum_Inproc/1  "VVMC_MSACtrlSta_enum"
  VVMC_MSACtrlSta_enum_Inproc/1 -> UnitConverter1072/1
  UnitConverter1072/1 -> VOUTP_MSACtrlSta_enum/1  "VOUTP_MSACtrlSta_enum"
  VVMC_APSCtrlAvail_flg/1 -> VVMC_APSCtrlAvail_flg_Inproc/1  "VVMC_APSCtrlAvail_flg"
  VVMC_APSCtrlAvail_flg_Inproc/1 -> UnitConverter1073/1
  UnitConverter1073/1 -> VOUTP_APSCtrlAvail_flg/1  "VOUTP_APSCtrlAvail_flg"
  VVMC_APSActive_flg/1 -> VVMC_APSActive_flg_Inproc/1  "VVMC_APSActive_flg"
  VVMC_APSActive_flg_Inproc/1 -> UnitConverter1074/1
  UnitConverter1074/1 -> VOUTP_APSActive_flg/1  "VOUTP_APSActive_flg"
  VVMC_APSStaSys_enum/1 -> VVMC_APSStaSys_enum_Inproc/1  "VVMC_APSStaSys_enum"
  VVMC_APSStaSys_enum_Inproc/1 -> UnitConverter1075/1
  UnitConverter1075/1 -> VOUTP_APSStaSys_enum/1  "VOUTP_APSStaSys_enum"
  VVMC_APSDecReqA_flg/1 -> VVMC_APSDecReqA_flg_Inproc/1  "VVMC_APSDecReqA_flg"
  VVMC_APSDecReqA_flg_Inproc/1 -> UnitConverter1076/1
  UnitConverter1076/1 -> VOUTP_APSDecReqA_flg/1  "VOUTP_APSDecReqA_flg"
  VVMC_APSDecReq_mps2/1 -> VVMC_APSDecReq_mps2_Inproc/1  "VVMC_APSDecReq_mps2"
  VVMC_APSDecReq_mps2_Inproc/1 -> UnitConverter1077/1
  UnitConverter1077/1 -> VOUTP_APSDecReq_mps2/1  "VOUTP_APSDecReq_mps2"
  VVMC_APSReq_enum/1 -> VVMC_APSReq_enum_Inproc/1  "VVMC_APSReq_enum"
  VVMC_APSReq_enum_Inproc/1 -> UnitConverter1078/1
  UnitConverter1078/1 -> VOUTP_APSReq_enum/1  "VOUTP_APSReq_enum"
  VVMC_LongAcc_Gps/1 -> VVMC_LongAcc_Gps_Inproc/1  "VVMC_LongAcc_Gps"
  VVMC_LongAcc_Gps_Inproc/1 -> UnitConverter1079/1
  UnitConverter1079/1 -> VOUTP_LongAcc_Gps/1  "VOUTP_LongAcc_Gps"
  VVMC_CCMSASpdWar_flg/1 -> VVMC_CCMSASpdWar_flg_Inproc/1  "VVMC_CCMSASpdWar_flg"
  VVMC_CCMSASpdWar_flg_Inproc/1 -> UnitConverter1080/1
  UnitConverter1080/1 -> VOUTP_CCMSASpdWar_flg/1  "VOUTP_CCMSASpdWar_flg"
  VVMC_IMUEnaCmd_flg/1 -> VVMC_IMUEnaCmd_flg_Inproc/1  "VVMC_IMUEnaCmd_flg"
  VVMC_IMUEnaCmd_flg_Inproc/1 -> UnitConverter1081/1
  UnitConverter1081/1 -> VOUTP_IMUEnaCmd_flg/1  "VOUTP_IMUEnaCmd_flg"
  VVMC_CAASCtrlAvail_flg/1 -> VVMC_CAASCtrlAvail_flg_Inproc/1  "VVMC_CAASCtrlAvail_flg"
  VVMC_CAASCtrlAvail_flg_Inproc/1 -> UnitConverter1082/1
  UnitConverter1082/1 -> VOUTP_CAASCtrlAvail_flg/1  "VOUTP_CAASCtrlAvail_flg"
  VVMC_CAASActive_flg/1 -> VVMC_CAASActive_flg_Inproc/1  "VVMC_CAASActive_flg"
  VVMC_CAASActive_flg_Inproc/1 -> UnitConverter1083/1
  UnitConverter1083/1 -> VOUTP_CAASActive_flg/1  "VOUTP_CAASActive_flg"
  VVMC_ExtraMSACtrlSta_enum/1 -> VVMC_ExtraMSACtrlSta_enum_Inproc/1  "VVMC_ExtraMSACtrlSta_enum"
  VVMC_ExtraMSACtrlSta_enum_Inproc/1 -> UnitConverter1084/1
  UnitConverter1084/1 -> VOUTP_ExtraMSACtrlSta_enum/1  "VOUTP_ExtraMSACtrlSta_enum"
  VVMC_CalibratedAccX_G/1 -> VVMC_CalibratedAccX_G_Inproc/1  "VVMC_CalibratedAccX_G"
  VVMC_CalibratedAccX_G_Inproc/1 -> UnitConverter1085/1
  UnitConverter1085/1 -> VOUTP_CalibratedAccX_G/1  "VOUTP_CalibratedAccX_G"
  VVMC_CalibratedAccY_G/1 -> VVMC_CalibratedAccY_G_Inproc/1  "VVMC_CalibratedAccY_G"
  VVMC_CalibratedAccY_G_Inproc/1 -> UnitConverter1086/1
  UnitConverter1086/1 -> VOUTP_CalibratedAccY_G/1  "VOUTP_CalibratedAccY_G"
  VVMC_CalibratedAccZ_G/1 -> VVMC_CalibratedAccZ_G_Inproc/1  "VVMC_CalibratedAccZ_G"
  VVMC_CalibratedAccZ_G_Inproc/1 -> UnitConverter1087/1
  UnitConverter1087/1 -> VOUTP_CalibratedAccZ_G/1  "VOUTP_CalibratedAccZ_G"
  VVMC_CalibratedGyroX_Dps/1 -> VVMC_CalibratedGyroX_Dps_Inproc/1  "VVMC_CalibratedGyroX_Dps"
  VVMC_CalibratedGyroX_Dps_Inproc/1 -> UnitConverter1088/1
  UnitConverter1088/1 -> VOUTP_CalibratedGyroX_Dps/1  "VOUTP_CalibratedGyroX_Dps"
  VVMC_CalibratedGyroY_Dps/1 -> VVMC_CalibratedGyroY_Dps_Inproc/1  "VVMC_CalibratedGyroY_Dps"
  VVMC_CalibratedGyroY_Dps_Inproc/1 -> UnitConverter1089/1
  UnitConverter1089/1 -> VOUTP_CalibratedGyroY_Dps/1  "VOUTP_CalibratedGyroY_Dps"
  VVMC_CalibratedGyroZ_Dps/1 -> VVMC_CalibratedGyroZ_Dps_Inproc/1  "VVMC_CalibratedGyroZ_Dps"
  VVMC_CalibratedGyroZ_Dps_Inproc/1 -> UnitConverter1090/1
  UnitConverter1090/1 -> VOUTP_CalibratedGyroZ_Dps/1  "VOUTP_CalibratedGyroZ_Dps"
  VVMC_FDCVMCAPSVRqEPSCtrl_flg/1 -> VVMC_FDCVMCAPSVRqEPSCtrl_flg_Inproc/1  "VVMC_FDCVMCAPSVRqEPSCtrl_flg"
  VVMC_FDCVMCAPSVRqEPSCtrl_flg_Inproc/1 -> UnitConverter1091/1
  UnitConverter1091/1 -> VOUTP_FDCVMCAPSVRqEPSCtrl_flg/1  "VOUTP_FDCVMCAPSVRqEPSCtrl_flg"
  VVMC_FDCVMCAPSAngleTarget_deg/1 -> VVMC_FDCVMCAPSAngleTarget_deg_Inproc/1  "VVMC_FDCVMCAPSAngleTarget_deg"
  VVMC_FDCVMCAPSAngleTarget_deg_Inproc/1 -> UnitConverter1092/1
  UnitConverter1092/1 -> VOUTP_FDCVMCAPSAngleTarget_deg/1  "VOUTP_FDCVMCAPSAngleTarget_deg"
  VVMC_FDCVMCAPSRqEPSCtrl_flg/1 -> VVMC_FDCVMCAPSRqEPSCtrl_flg_Inproc/1  "VVMC_FDCVMCAPSRqEPSCtrl_flg"
  VVMC_FDCVMCAPSRqEPSCtrl_flg_Inproc/1 -> UnitConverter1093/1
  UnitConverter1093/1 -> VOUTP_FDCVMCAPSRqEPSCtrl_flg/1  "VOUTP_FDCVMCAPSRqEPSCtrl_flg"
  VVMC_FDCVMCAngCtrlTqWtGn_pct/1 -> VVMC_FDCVMCAngCtrlTqWtGn_pct_Inproc/1  "VVMC_FDCVMCAngCtrlTqWtGn_pct"
  VVMC_FDCVMCAngCtrlTqWtGn_pct_Inproc/1 -> UnitConverter1094/1
  UnitConverter1094/1 -> VOUTP_FDCVMCAngCtrlTqWtGn_pct/1  "VOUTP_FDCVMCAngCtrlTqWtGn_pct"
  VVMC_FDCVMCDrInpTqBstAct_flg/1 -> VVMC_FDCVMCDrInpTqBstAct_flg_Inproc/1  "VVMC_FDCVMCDrInpTqBstAct_flg"
  VVMC_FDCVMCDrInpTqBstAct_flg_Inproc/1 -> UnitConverter1095/1
  UnitConverter1095/1 -> VOUTP_FDCVMCDrInpTqBstAct_flg/1  "VOUTP_FDCVMCDrInpTqBstAct_flg"
  VVMC_FDCVMCMaxAngCtrlOutTqLim_Nm/1 -> VVMC_FDCVMCMaxAngCtrlOutTqLim_Nm_Inproc/1  "VVMC_FDCVMCMaxAngCtrlOutTqLim_Nm"
  VVMC_FDCVMCMaxAngCtrlOutTqLim_Nm_Inproc/1 -> UnitConverter1096/1
  UnitConverter1096/1 -> VOUTP_FDCVMCMaxAngCtrlOutTqLim_Nm/1  "VOUTP_FDCVMCMaxAngCtrlOutTqLim_Nm"
  VVMC_FDCVMCDrInpTqBstGn_pct/1 -> VVMC_FDCVMCDrInpTqBstGn_pct_Inproc/1  "VVMC_FDCVMCDrInpTqBstGn_pct"
  VVMC_FDCVMCDrInpTqBstGn_pct_Inproc/1 -> UnitConverter1097/1
  UnitConverter1097/1 -> VOUTP_FDCVMCDrInpTqBstGn_pct/1  "VOUTP_FDCVMCDrInpTqBstGn_pct"
